simulink model "inga_Kapica"  (Simulink 7.8)
settings: Solver=ode45  StartTime=0.0  StopTime=inf  RelTol=1e-3
values from neighbouring files (symbols this model uses):
  x1 = -pi:0.3:3*pi    [inga.m]
  x2 = -2:0.3:2    [inga.m]
libraries: vrlib x3
settings Model: Creator=valaki  LastModifiedBy=valaki

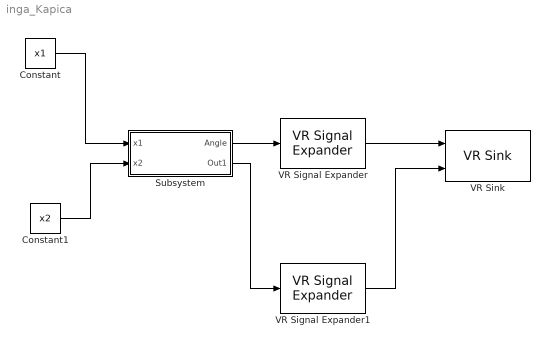
== system inga_Kapica ==
  Constant : Constant  Value=x1
  Constant1 : Constant  Value=x2
  Subsystem : Subsystem
  VR Signal Expander : vrlib/VR Signal Expander  outwidth=4  outidx=[4]
  VR Signal Expander1 : vrlib/VR Signal Expander  outwidth=3  outidx=[2]
  VR Sink : vrlib/VR Sink  SampleTime=0.1  ViewEnable=on  RemoteChange=off  RemoteView=off  FieldsWritten=Ball.rotation.4.1.1.double#Ball.translation.3.1.1.double  WorldFileName=C:\Users\valaki\Desktop\Pendulum_3D_Kapica.wrl  WorldDescription=Forced Damped Pendulum  AutoView=off  VideoDimensions=[]  AllowVariableSize=off
  wires:
  Constant/1 -> Subsystem/1(x1)
  Constant1/1 -> Subsystem/2(x2)
  Subsystem/1(Angle) -> VR Signal Expander/1
  VR Signal Expander/1 -> VR Sink/1
  Subsystem/2(Out1) -> VR Signal Expander1/1
  VR Signal Expander1/1 -> VR Sink/2

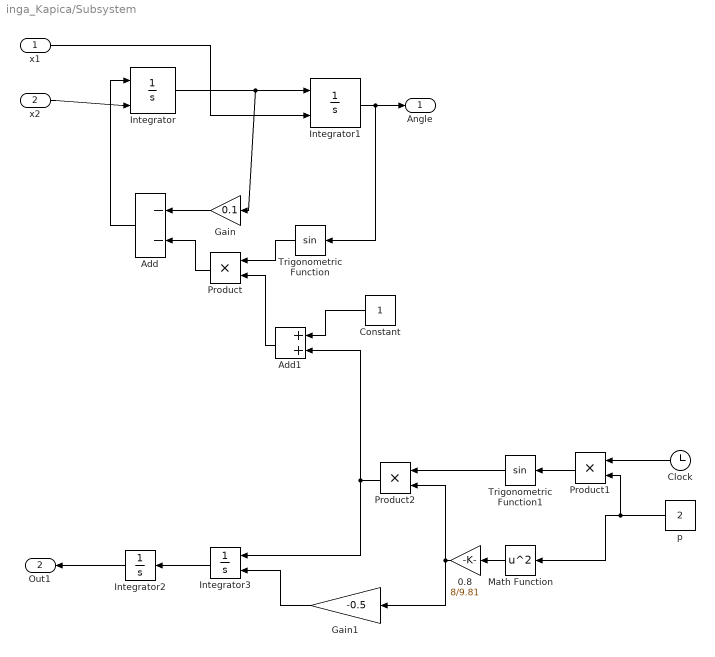
== system inga_Kapica/Subsystem ==
  x1 : Inport
  x2 : Inport  Port=2
  0.8 : Gain  Gain=8/9.81
  Add : Sum  Inputs=--
  Add1 : Sum
  Clock : Clock
  Constant : Constant
  Gain : Gain  Gain=0.1
  Gain1 : Gain  Gain=-0.5
  Integrator : Integrator  InitialConditionSource=external
  Integrator1 : Integrator  InitialConditionSource=external
  Integrator2 : Integrator
  Integrator3 : Integrator  InitialConditionSource=external
  Math Function : Math  Operator=square  SaturateOnIntegerOverflow=on
  Product : Product  RndMeth=Zero
  Product1 : Product  RndMeth=Zero
  Product2 : Product  RndMeth=Zero
  Trigonometric Function : Trigonometry
  Trigonometric Function1 : Trigonometry
  p : Constant  Value=2
  Angle : Outport
  Out1 : Outport  Port=2
  wires:
  x2/1 -> Integrator/2
  Integrator/1 -> Integrator1/1, Gain/1
  x1/1 -> Integrator1/2
  Integrator1/1 -> Angle/1, Trigonometric Function/1
  Add/1 -> Integrator/1
  Gain/1 -> Add/1
  Product/1 -> Add/2
  Trigonometric Function/1 -> Product/1
  Constant/1 -> Add1/1
  Add1/1 -> Product/2
  p/1 -> Math Function/1, Product1/2
  Trigonometric Function1/1 -> Product2/1
  Product1/1 -> Trigonometric Function1/1
  Clock/1 -> Product1/1
  Product2/1 -> Add1/2, Integrator3/1
  Math Function/1 -> 0.8/1
  0.8/1 -> Product2/2, Gain1/1
  Integrator2/1 -> Out1/1
  Integrator3/1 -> Integrator2/1
  Gain1/1 -> Integrator3/2
